simulink model "x0210_GS (3)"  (R2024a)
settings: Solver=VariableStepAuto  StartTime=0.0  StopTime=10.0  RelTol=1e-3
values from neighbouring files (symbols this model uses):
  actuator_delay = 1    [matlab.mat]    (also in untitled.m = single(1))
  gear_1_lower_threshold = 5    [matlab.mat]    (also in untitled.m = single(5))
  gear_1_upper_threshold = 900    [matlab.mat]    (also in untitled.m = single(900))
  gear_2_lower_threshold = 5    [matlab.mat]    (also in untitled.m = single(5))
  gear_2_upper_threshold = 450    [matlab.mat]    (also in untitled.m = single(450))
  speed_tolerance_diseng_rpm = 10    [matlab.mat]    (also in untitled.m = single(10))
  speed_tolerance_rpm = 10    [matlab.mat]    (also in untitled.m = single(10))
  sync_delay = 3    [matlab.mat]    (also in untitled.m = single(3))
settings Model: TunableVars=gear_1_lower_threshold,gear_1_upper_threshold,gear_2_lower_threshold,gear_2_upper_threshold,speed_tolerance_diseng_rpm,speed_tolerance_rpm,sync_delay,actuator_delay  TunableVarsStorageClass=Auto,Auto,Auto,Auto,Auto,Auto,Auto,Auto  TunableVarsTypeQualifier=,,,,,,,  Creator=kwsha  LastModifiedBy=ibanagar22
settings ConfigComp: PLC_TargetIDE=codesys35  PLC_MultiTBSigbuilderTimeRange=off  PLC_FoldFBCallOutputVar=off  PLC_RemoveUnusedSSMethodCallArguments=off  PLC_UseCallOutputArgSyntax=off  PLC_EnableUnsignedAndDoubleTypes=off  PLC_EnableUDTSplitting=off  PLC_MaxFieldsInUDT=500  PLC_InlineEnumCastFunction=off

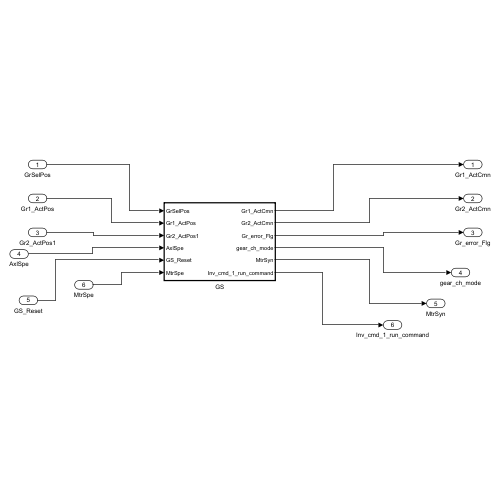
[thumbnail: Simulink's stored preview of the top-level diagram]
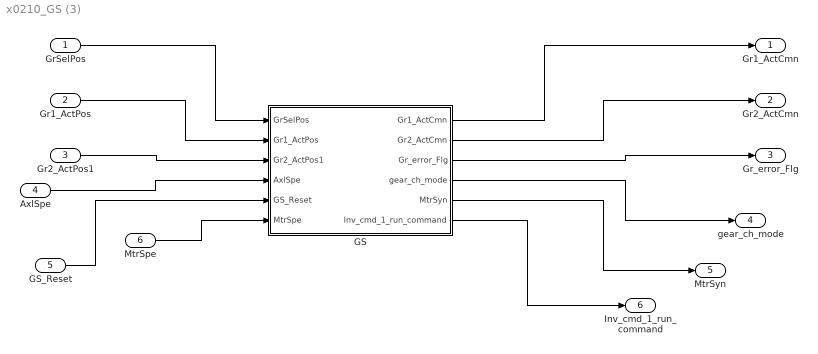
== system x0210_GS (3) ==
  GrSelPos : Inport
  Gr1_ActPos : Inport  Port=2
  Gr2_ActPos1 : Inport  Port=3
  AxlSpe : Inport  Port=4  Unit=rpm
  GS_Reset : Inport  Port=5
  MtrSpe : Inport  Port=6  Unit=rpm
  GS : Subsystem  TreatAsAtomicUnit=on
  Gr1_ActCmn : Outport
  Gr2_ActCmn : Outport  Port=2
  Gr_error_Flg : Outport  Port=3
  gear_ch_mode : Outport  Port=4
  MtrSyn : Outport  Port=5
  Inv_cmd_1_run_command : Outport  Port=6
  wires:
  GrSelPos/1 -> GS/1(GrSelPos)
  Gr1_ActPos/1 -> GS/2(Gr1_ActPos)
  Gr2_ActPos1/1 -> GS/3(Gr2_ActPos1)
  AxlSpe/1 -> GS/4(AxlSpe)
  GS_Reset/1 -> GS/5(GS_Reset)
  MtrSpe/1 -> GS/6(MtrSpe)
  GS/1(Gr1_ActCmn) -> Gr1_ActCmn/1
  GS/2(Gr2_ActCmn) -> Gr2_ActCmn/1
  GS/3(Gr_error_Flg) -> Gr_error_Flg/1
  GS/4(gear_ch_mode) -> gear_ch_mode/1
  GS/5(MtrSyn) -> MtrSyn/1
  GS/6(Inv_cmd_1_run_command) -> Inv_cmd_1_run_command/1

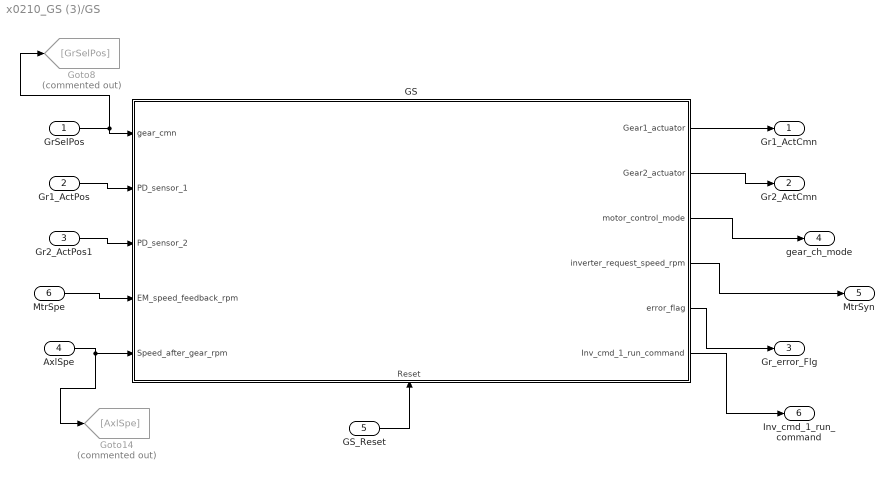
== system x0210_GS (3)/GS ==
  GrSelPos : Inport
  Gr1_ActPos : Inport  Port=2  OutDataTypeStr=boolean
  Gr2_ActPos1 : Inport  Port=3  OutDataTypeStr=boolean
  AxlSpe : Inport  Port=4  Unit=rpm
  GS_Reset : Inport  Port=5
  MtrSpe : Inport  Port=6  Unit=rpm
  GS : Stateflow chart  TreatAsAtomicUnit=on
      settings: PortSchema="{\"entries\":[{\"content\":{\"sides\":[{\"content\":{\"connectorIds\":[\"In1\",\"In2\",\"In3\",\"In5\",\"In6\"]},\"type\":\"ConnectorPlacement.EquallySpacedRectSide\",\"uuid\":\"d6e14f2c-3aed-42e8-8853-b3bc1cd3db5e\"},{\"content\":{\"connectorIds\":[\"Out1\",\"Out2\",\"Out3\",\"Out4\",\"Out5\",\"Out6\"],\"side\":\"RIGHT\"},\"type\":\"ConnectorPlacement.EquallySpacedRectSide\",\"uuid\":\"2ce6c22a-ad7c-4e64-9a73-673441d8f644\"},{\"content\":{\"side\":\"TOP\"},\"type\":\"ConnectorPlacement.EquallySpacedRectSide\",\"uuid\":\"cfc594f6-626d-4d59-9903-7d8b8221362b\"},{\"content\":{\"connectorIds\":[\"In4\"],\"side\":\"BOTTOM\"},\"type\":\"ConnectorPlacement.EquallySpacedRectSide\",\"uuid\":\"dc010bbd-c54a-4109-850f-255182d54186\"}]},\"type\":\"ConnectorPlacement.EquallySpacedConnector\",\"uuid\":\"7594eabf-140f-4880-b985-77459c5dbf53\"}],\"packageUris\":[\"http://schema.mathworks.com/mf0/Connector/R2020b\"],\"version\":\"1.0\"}"
  Goto14 : Goto  Commented=on  GotoTag=AxlSpe
  Goto8 : Goto  Commented=on  GotoTag=GrSelPos
  Gr1_ActCmn : Outport
  Gr2_ActCmn : Outport  Port=2
  Gr_error_Flg : Outport  Port=3
  gear_ch_mode : Outport  Port=4
  MtrSyn : Outport  Port=5
  Inv_cmd_1_run_command : Outport  Port=6
  wires:
  GS/5(error_flag) -> Gr_error_Flg/1
  AxlSpe/1 -> Goto14/1, GS/6(Speed_after_gear_rpm)
  Gr2_ActPos1/1 -> GS/3(PD_sensor_2)
  MtrSpe/1 -> GS/5(EM_speed_feedback_rpm)
  GS/2(Gear2_actuator) -> Gr2_ActCmn/1
  GrSelPos/1 -> Goto8/1, GS/1(gear_cmn)
  GS_Reset/1 -> GS/4(Reset)
  GS/1(Gear1_actuator) -> Gr1_ActCmn/1
  Gr1_ActPos/1 -> GS/2(PD_sensor_1)
  GS/4(inverter_request_speed_rpm) -> MtrSyn/1
  GS/3(motor_control_mode) -> gear_ch_mode/1
  GS/6(Inv_cmd_1_run_command) -> Inv_cmd_1_run_command/1

== stateflow chart x0210_GS (3)/GS/GS ==
  state Sync
    %if not match the speed after 5 sec, go to the safe mode
    %if not gear disengaged,go to safe mode
    % circuit opens when the gear is engaged (engaged =0)
    %PD_sensor - Position Detection Sensor
    %EM_feedback - 1 -150 / 2-70
    entry:
    Inv_cmd_1_run_command=1;
    safe_mode_trigger = 0;
    during:
    if gear_cmn == 1
    gear_rotation_speed_1_rpm = Speed_after_gear_rpm*2.31;
    if gear_1_lower_threshold <= gear_rotation_speed_1_rpm &&  gear_rotation_speed_1_rpm <= gear_1_upper_threshold
    motor_control_mode = true;
    inverter_request_speed_rpm = gear_rotation_speed_1_rpm - 10;
    else safe_mode_trigger =1;
    end
    elseif gear_cmn == 2
    gear_rotation_speed_2_rpm = Speed_after_gear_rpm*1.011;
    if gear_2_lower_threshold <= gear_rotation_speed_2_rpm && gear_rotation_speed_2_rpm <= gear_2_upper_threshold
    motor_control_mode = true;
    inverter_request_speed_rpm = gear_rotation_speed_2_rpm -10;
    else safe_mode_trigger =1;
    end
    end
  state Eng_gear1
    entry:
    during:
    Inv_cmd_1_run_command=1;
    Gear1_actuator=true;
    Gear2_actuator=false;
    motor_control_mode = false;
    exit:
    Engage_gear_1=1;
    Engage_gear_2=0;
  state Engagging_gear_one
    during:
    inverter_request_speed_rpm = inverter_request_speed_rpm;
    Gear1_actuator=true;
    Gear2_actuator=false;
    Inv_cmd_1_run_command=1;
    exit:
    Gear1_actuator=true;
    Gear2_actuator=false;
  state disengaging_gear
    entry:
    Inv_cmd_1_run_command=1;
    motor_control_mode = true;
    during:
    if Engage_gear_1 ==1
    inverter_request_speed_rpm = Speed_after_gear_rpm*2.31;
    if abs(EM_speed_feedback_rpm - inverter_request_speed_rpm) <= speed_tolerance_diseng_rpm
    Gear1_actuator=false;
    end
    end
    if Engage_gear_2 ==1
    inverter_request_speed_rpm = Speed_after_gear_rpm*1.011;
    if abs(EM_speed_feedback_rpm - inverter_request_speed_rpm) <= speed_tolerance_diseng_rpm
    Gear2_actuator=false;
    end
    end
    exit:
    Engage_gear_1=0;
    Engage_gear_2=0;
  state Nutral
    entry:
    Inv_cmd_1_run_command=1;
    Gear1_actuator=false;
    Gear2_actuator=false;
    during:
    motor_control_mode = false;
    exit:
    Engage_gear_1=0;
    Engage_gear_2=0;
  state Detecting_gear
    entry:
    safe_mode_trigger = 0;
    during:
    if PD_sensor_1 == true || PD_sensor_2 == true
    safe_mode_trigger = 1;
    else safe_mode_trigger = 0;
    end
  state Eng_gear2
    entry:
    during:
    Inv_cmd_1_run_command=1;
    Gear1_actuator=false;
    Gear2_actuator=true;
    motor_control_mode = false;
    %if abs(EM_speed_feedback_rpm - inverter_request_speed_rpm)>speed_tolerance_rpm
    %  safe_mode_trigger=1;
    %end
    exit:
    Engage_gear_1=0;
    Engage_gear_2=1;
  state Engagging_gear_two
    during:
    Inv_cmd_1_run_command=1;
    inverter_request_speed_rpm = inverter_request_speed_rpm;
    Gear1_actuator=false;
    Gear2_actuator=true;
    exit:
    Gear1_actuator=false;
    Gear2_actuator=true;
  state Safe_mode
    during:
    Engage_gear_1 = 0;
    Engage_gear_2 = 0;
    Gear1_actuator = false;
    Gear2_actuator = false;
    motor_control_mode = false;
    error_flag=true;
    exit:
    safe_mode_trigger = 0;
    error_flag=false;
  Nutral -> Sync : [gear_cmn==1 || gear_cmn==2 ]
  Sync -> (junction 125) [order 2] : [after(sync_delay,sec)]
  disengaging_gear -> Sync [order 2] : [PD_sensor_1==false && PD_sensor_2==false  ]
  Sync -> Safe_mode [order 1] : [safe_mode_trigger == 1 || after(6, sec)]
  Engagging_gear_one -> Eng_gear1 : [ PD_sensor_1==true && after(actuator_delay,sec)]{Inv_cmd_1_run_command=0}
  Eng_gear1 -> disengaging_gear [order 1] : [gear_cmn ~= 1]
  Detecting_gear -> Eng_gear1 [order 3] : [PD_sensor_1==true && PD_sensor_2==false]
  (junction 125) -> Engagging_gear_one [order 1] : [abs(EM_speed_feedback_rpm - inverter_request_speed_rpm) < speed_tolerance_rpm && gear_cmn==1]
  Eng_gear1 -> Safe_mode [order 2] : [safe_mode_trigger == 1]
  (junction 125) -> Engagging_gear_two [order 2] : [abs(EM_speed_feedback_rpm - inverter_request_speed_rpm) < speed_tolerance_rpm && gear_cmn==2]
  (default) -> Detecting_gear
  disengaging_gear -> Nutral [order 1] : [gear_cmn==0 && PD_sensor_1==false && PD_sensor_2 ==false]
  Detecting_gear -> Nutral [order 2] : [PD_sensor_1==false && PD_sensor_2==false]
  Eng_gear2 -> disengaging_gear [order 1] : [gear_cmn~=2]
  disengaging_gear -> Safe_mode [order 3] : after(5,sec)
  Detecting_gear -> Safe_mode [order 1] : [safe_mode_trigger == 1]
  Safe_mode -> Detecting_gear : [Reset==true]%user input to reset
  Detecting_gear -> Eng_gear2 [order 4] : [PD_sensor_1==false && PD_sensor_2==true]
  Eng_gear2 -> Safe_mode [order 2] : [safe_mode_trigger == 1]
  Engagging_gear_two -> Eng_gear2 : [ PD_sensor_2==true && after(actuator_delay,sec)]{Inv_cmd_1_run_command=0;}
  data: Gear1_actuator output boolean; Gear2_actuator output boolean; gear_cmn input uint8; motor_control_mode output boolean; PD_sensor_1 input; PD_sensor_2 input; Engage_gear_1 local; Engage_gear_2 local; safe_mode_trigger local; Reset input boolean; EM_speed_feedback_rpm input; inverter_request_speed_rpm output; Speed_after_gear_rpm input; gear_rotation_speed_2_rpm local; gear_rotation_speed_1_rpm local; error_flag output boolean; speed_tolerance_rpm parameter; gear_1_lower_threshold parameter; gear_2_upper_threshold parameter; gear_2_lower_threshold parameter; gear_1_upper_threshold parameter; speed_tolerance_diseng_rpm parameter; actuator_delay parameter; sync_delay parameter; Inv_cmd_1_run_command output
